simulink model "Expriment_Pose"  (R2014a)
settings: Solver=FixedStepDiscrete  SolverMode=SingleTasking  StartTime=0.0  StopTime=inf  FixedStep=0.01  RelTol=1e-3
PostLoadFcn:
  | h_RPStest = RPStest;
model workspace (MAT data in the model file):
  gtest = 0
undefined symbols (not defined in the file or in its folder): avert, avert_freq_factor, avert_gaze_dirs_chance, avert_gaze_duration_factor, avert_head_frequency_factor, avert_head_speed, BML, BML1, BML2, bmlsL, bmlsM, bodyBusyFlag, clock, emotion_amount_factor, faceBusyFlag, fileID, GAZE_WIN, gazing, mut_freq_factor, mutual_gaze_duration_factor, P, pose_cat_chance, pose_chanc_factor, pose_chance_factor, pose_frequency_factor, pose_lean, pose_lean_flag, pose_speed, pose_twitch, pr, serial, STATE_BEFORE, STATE_GO, STATE_OVER, STATE_READY, Stateflow
libraries: simulink x24, instrumentlib x6, lib_affectiveChar_behavior x2, realtime_pacer_lib x2, lib_affectiveChar_input x1
(part 7 of 7)

== stateflow chart Expriment_Pose/CharacterControl/facialExpression_Controller ==
  state subSmile [parallel]
    settings: executionOrder=1
    state stateInitial
      entry: avert=1; gameState=14;
      n=encStr2Arr(' ');bmlsM=[n n n n n];newBmlsM=[n n n n n];
    state stateCheckSmile
    state gazeCamera
      entry:  [P,BMLM]= smileTable(2) ;avert=0;
      newBmlsM=insertQueue(bmlsM,BMLM);
      bmlsM=newBmlsM;
    state wait
    state checkP
      entry:  [P,BMLM]=  smileTable(1) ;
      newBmlsM=insertQueue(bmlsM,BMLM);
      bmlsM=newBmlsM;
    (default) -> stateInitial
    stateInitial -> stateCheckSmile : [gameState==20]
    stateCheckSmile -> stateCheckSmile [order 2]
    gazeCamera -> stateCheckSmile [order 2] : after(1,secs)[isSmiling~=1]
    wait -> stateCheckSmile : after(10,secs)
    stateCheckSmile -> gazeCamera [order 1] : [[isSmiling==1]&[ gameState~= STATE_GO]&[ gameState~= STATE_READY]]
    checkP -> wait
    gazeCamera -> checkP [order 1] : after(1,secs)[isSmiling==1]
  note: SMILE_DUER=10 seceonds
  note: check if still isSmiling is true works as a buffer to remove the smiles that last ony 1 sec (system errors).
  state subFacial [parallel]
    settings: executionOrder=2
    state stateFacialExpression
      entry:
      emotion_amount_factor =set_AU_Amount(inA,inV,personality);
      BMLl=cmdBML_AU_VA(emotion_amount_factor);
      newBmlsL=insertQueueLow(bmlsL,BMLl); bmlsL=newBmlsL;
    state initial
    state wait3
    (default) -> initial
    initial -> stateFacialExpression : [gameState==20]
    wait3 -> stateFacialExpression : after(7,secs)
    stateFacialExpression -> wait3
  data: bmls function_input double size=[1000,5]; myBML function_input double size=[1000,1]; newBmls function_output double size=[1000,5]; bmls function_input double size=[1000,5]; myBML function_input double size=[1000,1]; newBmls function_output double size=[1000,5]; bmlID function_input double; p function_output double size=1; poseBML function_output double size=[1000,1]; bmlID function_input double; p function_output double size=1; poseBML function_output double size=[1000,1]; eAmountFactor function_output double size=[1,11]; arousal function_input double size=1; valence function_input double size=1; inPersonality function_input double size=1; smileN local double size=1; isSmiling input double size=1 =0; avert data_store_memory =0; gazing data_store_memory size=2; GAZE_WIN data_store_memory size=2; BML data_store_memory size=[256,1]; P data_store_memory; fileID local double size=1; gameState output double; STATE_GO data_store_memory; STATE_READY data_store_memory; STATE_BEFORE data_store_memory; newBmlsM local double size=[1000,5]; bmlsM data_store_memory size=[256,1]; BMLM local double size=[1000,1]; n local; personality input double size=1; internalE input double size=1; au local; emotion_amount_factor data_store_memory; aChange input boolean size=1; au_i local double size=1; au_L local double size=1; emoDisp local; bmlsL data_store_memory size=[256,1]; BMLl local double size=[1000,1]; newBmlsL local double size=[1000,5]; emotion_amount_custom input double size=1; inA input double size=1; inV input double size=1; vChange input boolean size=1
  events: secs input RISING_EDGE_EVENT
  function newBmls =insertQueue(bmls,myBML):
    | function newBmls =insertQueue(bmls,myBML)
    |     full=1;
    |     t=encStr2Arr(' ');
    |     newBmls=[t t t t t];
    |     for i = 1:5
    |         if (isequal(bmls(:,i),t))
    |             %add to end of the queue where its empty
    |             bmls(:,i)=myBML;
    |             full=0;
    |             break
    |         end
    |     end
    |     if(full~=0)
    |             %if queue full, shift all elements to left which removes the first one, then add to end
    |             bmls(:,1)= bmls(:,2);
    |             bmls(:,2)= bmls(:,3);
    |             bmls(:,3)= bmls(:,4);
    |             bmls(:,5)=myBML;
    |     end
    |     newBmls=bmls;
  function newBmls =insertQueueLow(bmls,myBML):
    | function newBmls =insertQueueLow(bmls,myBML)
    |     full=1;
    |     t=encStr2Arr(' ');
    |     newBmls=[t t t t t];
    |     for i = 1:5
    |         if (isequal(bmls(:,i),t))
    |             %add to end of the queue where its empty
    |             bmls(:,i)=myBML;
    |             full=0;
    |             break
    |         end
    |     end
    |     if(full~=0)
    |             %if queue full, shift all elements to left which removes the first one, then add to end
    |             bmls(:,1)= bmls(:,2);
    |             bmls(:,2)= bmls(:,3);
    |             bmls(:,3)= bmls(:,4);
    |             bmls(:,5)=myBML;
    |     end
    |     newBmls=bmls;
  function [p,poseBML] = smileTable(bmlID):
    | function [p,poseBML] = smileTable(bmlID)
    | 
    | aVarTruthTableCondition_1 = false;
    | aVarTruthTableCondition_2 = false;
    | 
    | 
    | % smile
    | 
    | aVarTruthTableCondition_1 = logical(bmlID==1);
    | 
    | % headN
    | 
    | aVarTruthTableCondition_2 = logical(bmlID==2);
    | 
    | if (aVarTruthTableCondition_1)
    |     aFcnTruthTableAction_1();
    | elseif (aVarTruthTableCondition_2)
    |     aFcnTruthTableAction_2();
    | else % Default
    |     aFcnTruthTableAction_1();
    | end
    | 
    | function aFcnTruthTableAction_1()
    | 
    | % smile
    | 
    | poseBML=encStr2Arr('<?xml version="1.0"?><act><bml><face amount="1" au="12" side="BOTH" start="0" stroke="2" relax="3" end="4" type="facs"/><face amount="0.3" au="6" side="BOTH" start="0" stroke="2" relax="3" end="4" type="facs"/></bml></act>');p=3;
    | 
    | function aFcnTruthTableAction_2()
    | 
    | % headNeutralBrow
    | 
    | poseBML=encStr2Arr('<?xml version="1.0" ?><act><bml><gaze target="gazeTarget" start="0" end="5" sbm:time-hint="1.5"/></bml></act>');p=3;
    | 
    | function aFcnTruthTableAction_3()
    | 
    | % smileBrow
    | 
    | poseBML=encStr2Arr('<?xml version="1.0"?><act><bml><face amount="0.1" au="1" side="BOTH" start="0" stroke="2" relax="4" end="6" type="facs"/><face amount="0.1" au="2" side="BOTH" start="0" stroke="2" relax="4" end="6" type="facs"/></bml></act>');p=3;
  function [p,poseBML] = facialExpr(bmlID):
    | function [p,poseBML] = facialExpr(bmlID)
    | 
    | aVarTruthTableCondition_1 = false;
    | aVarTruthTableCondition_2 = false;
    | 
    | 
    | % smile
    | 
    | aVarTruthTableCondition_1 = logical(bmlID==1);
    | 
    | % headN
    | 
    | aVarTruthTableCondition_2 = logical(bmlID==2);
    | 
    | if (aVarTruthTableCondition_1)
    |     aFcnTruthTableAction_1();
    | elseif (aVarTruthTableCondition_2)
    |     aFcnTruthTableAction_2();
    | else % Default
    |     aFcnTruthTableAction_1();
    | end
    | 
    | function aFcnTruthTableAction_1()
    | 
    | % smile
    | 
    | poseBML=encStr2Arr('<?xml version="1.0"?><act><bml><face amount="1" au="12" side="BOTH" start="0" stroke="10" relax="70" end="100" type="facs"/><face amount="0.3" au="6" side="BOTH" start="0" stroke="10" relax="70" end="100" type="facs"/></bml></act>');p=3;
    | 
    | function aFcnTruthTableAction_2()
    | 
    | % headNeutralBrow
    | 
    | poseBML=encStr2Arr('<?xml version="1.0" ?><act><bml><gaze target="gazeTarget" start="0" end="5" sbm:time-hint="1.5"/></bml></act>');p=3;
    | 
    | function aFcnTruthTableAction_3()
    | 
    | % smileBrow
    | 
    | poseBML=encStr2Arr('<?xml version="1.0"?><act><bml><face amount="0.1" au="1" side="BOTH" start="0" stroke="2" relax="4" end="6" type="facs"/><face amount="0.1" au="2" side="BOTH" start="0" stroke="2" relax="4" end="6" type="facs"/></bml></act>');p=3;
  function eAmountFactor  =set_AU_Amount(arousal,valence,inPersonality):
    | function eAmountFactor  =set_AU_Amount(arousal,valence,inPersonality)
    | %     15-12-2015, PAD drivern facial expr simul, Grammer data to map AU and VA
    | %     fprintf('VA: %0.0f,%0.0f\r\n',arousal,valence);
    | %     scale
    | %     p = valence * (20/9)  - 10;
    | %     a = arousal * (20/9)  - 10;
    | 
    |     p=valence;a=arousal;
    |     all_AUs=[1,2,4,5,6, 7,12,26,45,10, 25];eAmountFactor=[0,0,0,0,0, 0,0,0,0,0, 0];
    |     for c=1:11
    |         eAmountFactor(1)=0.003*p-0.002*a;  %1,-0.002*a
    |         eAmountFactor(2)=-0.002*p+0.010*a; %2,+0.010*a
    | %         eAmountFactor(12)=-0.016*p+0.034*a; %27 moth open stretch
    |         eAmountFactor(8)=-0.002*p+0.023*a;  %26,-0.002*p+0.049*a
    |         eAmountFactor(5)=-0.008*p+0.009*a;  %6
    |         
    | %         eAmountFactor(13)=0.002*p+0.004*a; %18 lip Puckerer, W 0.3=101
    | %         eAmountFactor(14)=0.007*p+0.025*a; %22 lip fumeler, ShCh 0.5=102       
    | %         eAmountFactor(15)=0.003*p+0.009*a; %14 dimpler FV+PBM 0.5=103
    | %         eAmountFactor(16)=0.003*p+0.009*a; %14 dimpler FV+PBM 0.5=103
    | %         eAmountFactor=-0.010*p+0.017*a;  %17 chin raiser
    | 
    |         eAmountFactor(10)=-0.020*p+0.020*a;  %10 upper lip raiser,-0.053*p+0.026*a
    |         eAmountFactor(4)=-0.003*p+0.032*a; %5 upper lid raiser
    |         eAmountFactor(9)=-0.011*p-0.011*a; %eye closed, 45 instead of 43,-0.021*p-0.037*a
    |         eAmountFactor(3)=-0.036*p+0.022*a; %4 brow lowerer
    | %       eAmountFactor=-0.008*p+0.006*a;    %9 nose wrikler ,10
    | %       eAmountFactor=-0.004*p+0.004*a;    %39?
    | %       eAmountFactor=-0.010*p+0.008*a;    %38?
    | 
    |         eAmountFactor(11)=-0.011*p+0.023*a;%25 lip open,-0.023*p+0.058*a
    | %       eAmountFactor(17)=-0.004*p-0.003*a;    %24 lip pressor, PBM =104       
    | %       eAmountFactor(18)=-0.011*p+0.009*a;    %23 lip tightner PBM0.2 + W0.6=105
    | %       eAmountFactor(19)=-0.011*p+0.009*a;    %23 lip tightner PBM0.2 + W0.6=105
    | 
    | %       eAmountFactor=-0.004*p+0.003*a;    %19?
    | 
    | %       eAmountFactor(20)=0.039*p+0.015*a;  %13 cheek puffer, W 0.3 =106
    |         
    |         eAmountFactor(6)=-0.005*p-0.001*a; %7  Lid Tightener
    |         eAmountFactor(7)=0.057*p+0.009*a;  %12 Lip Corner Puller
    |     %   eAmountFactor=-0.008*p+0.009*a;    %11 Nasolabial Deepener
    |     %   eAmountFactor=-0.046*p-0.002*a;    %15 Lip Corner Depressor
    |     %   eAmountFactor=-0.014*p+0.016*a;    %16 Lower Lip Depressor
    |     %   eAmountFactor(20)=-0.026*p+0.010*a;%20 lip stretch
    |         
    |         eAmountFactor=eAmountFactor/6; %scale
    |         if(inPersonality==2 || inPersonality==4)%introvert
    |             eAmountFactor=eAmountFactor/1.3; % divide by 4/3
    |         end
    |     end

== stateflow chart Expriment_Pose/GazeFollowSubsystem/reactiveGaze/createGazePawn ==
  state sendBML(In1) [function]
  state sendSBM(In2) [function]
  state stateCreatePawn
    entry:
    sendSBM( encStr2Arr( 'gt = scene.createPawn("gazeTarget")' ) );
    sendBML(encStr2Arr('<?xml version="1.0" ?><act><bml><gaze sbm:joint-range="EYES BACK" target="gazeTarget"/></bml></act>'));
  (default) -> stateCreatePawn
  data: In1 function_input double size=[1000 1]; In2 function_input double size=[1000 1]

== matlab function Expriment_Pose/randomArray/makleArray ==
  data: r1 input; y output double size=[1,25]; r2 input; r3 input; r4 input; r5 input; r6 input; r7 input; r8 input; r9 input; r10 input; r11 input; r12 input; r13 input; r14 input; r15 input; r16 input; r17 input; r18 input; r19 input; r20 input; r21 input; r22 input; r23 input; r24 input; r25 input
function y = fcn(r1,r2,r3,r4,r5,r6,r7,r8,r9,r10,r11,r12,r13,r14,r15,r16, r17, r18, r19,r20,r21,r22,r23,r24,r25)
%#codegen
y=[0,0,0,0,0,0,0,0,0,0,0,0,0,0,0,0,0,0,0,0,0,0,0,0,0];
y(:,1) = floor(r1);
y(:,2) = floor(r2);
y(:,3) = floor(r3);
y(:,4) = floor(r4);
y(:,5) = floor(r5);
y(:,6) = floor(r6);
y(:,7) = floor(r7);
y(:,8) = floor(r8);
y(:,9) = floor(r9);
y(:,10) = floor(r10);
y(:,11) = floor(r11);
y(:,12) = floor(r12);
y(:,13) = floor(r13);
y(:,14) = floor(r14);
y(:,15) = floor(r15);
y(:,16) = floor(r16);
y(:,17) = floor(r17);
y(:,18) = floor(r18);
y(:,19) = floor(r19);
y(:,20) = floor(r20);
y(:,21) = floor(r21);
y(:,22) = floor(r22);
y(:,23) = floor(r23);
y(:,24) = floor(r24);
y(:,25) = floor(r25);

== matlab function Expriment_Pose/facialExpr/checkNeutral ==
  data: notNeutral output double size=1; e input
function notNeutral = fcn(e)
%#codegen

if(e~=6)
    notNeutral=1;
else
    notNeutral=0;
end

== stateflow chart Expriment_Pose/CharacterControl/wave_Controller ==
  state init
    entry: STATE_OVER=3;
    STATE_BEFORE=4;
    gameState=14;
    rFlag=0;lFlag=0;bFlag=0;
    n=encStr2Arr(' ');bmlsM=[n n n n n];
    newBmlsM=[n n n n n];
  state waveRightHand
    entry: [P,BMLM]= wavePoseBradTable(1+animNum);
    rFlag=1;
    newBmlsM=insertQueue(bmlsM,BMLM);
    bmlsM=newBmlsM;
  state gazeCamera
    entry: [P,BMLM]= wavePoseBradTable(8);
    avert=0;
    newBmlsM=insertQueue(bmlsM,BMLM);
    bmlsM=newBmlsM;
  state wave
    entry: animNum =setPersonalityParams(personality);
  state waveLeftHand
    entry:
    [P,BMLM]= wavePoseBradTable(animNum);
    lFlag=1;
    newBmlsM=insertQueue(bmlsM,BMLM);
    bmlsM=newBmlsM;
  state gazeCamera1
    entry: [P,BMLM]= wavePoseBradTable(8);
    avert=0;
    newBmlsM=insertQueue(bmlsM,BMLM);
    bmlsM=newBmlsM;
  note: if introvert 50% chance of introvertWave(poseN=7)
  note: else(extrovert)
  state gazeCamera2
    entry: [P,BMLM]= wavePoseBradTable(8);
    avert=0;
    newBmlsM=insertQueue(bmlsM,BMLM);
    bmlsM=newBmlsM;
  state waveBothHands
    entry: [P,BMLM]= wavePoseBradTable(3+animNum);
    bFlag=1;
    newBmlsM=insertQueue(bmlsM,BMLM);
    bmlsM=newBmlsM;
  note: Problem with procedural behaviors (you can not give duration and they stay in that pose untill new bml comes so they dont return to idle)
      | we want the agent to gaze at user for the period of waving.If new idle gaze BML comes, agent averts gaze or head before wave finished. Gaze is procedural (gazes at the point till new gaze bml is recieved so it does not automatically return to idle pose) so we can not give duration of gaze in the BML. The only way to avoid avert during wave is to make sure thre is no idle gaze bmls during the wave; which makes sense considering the gaze does not avert(idle) when you are attending something.
      | prioritizing does not solve this because avertGaze comes right after gazeCamera and wave. We also can not delay after high priorities because sometime several high priorities should happen right after eachother.
  waveBothHands -> wave : after(5,secs)
  waveRightHand -> wave : after(5,secs)
  waveLeftHand -> wave : after(5,secs)
  (default) -> init
  init -> wave
  (junction 55) -> waveRightHand [order 2]
  gazeCamera -> waveRightHand : after(2,secs)
  wave -> (junction 55) [order 4] : [[handUp==1]&[rFlag==0]]{ lFlag=0;bFlag=0;}
  (junction 55) -> gazeCamera [order 1] : [avert==1]
  wave -> wave [order 1] : after(10,secs){ rFlag=0;lFlag=0;bFlag=0;}
  wave -> (junction 59) [order 3] : [[handUp==3]&[bFlag==0]]{ rFlag=0;lFlag=0;}
  wave -> (junction 58) [order 2] : [[handUp==2]&[lFlag==0]]{ rFlag=0;bFlag=0;}
  (junction 82) -> waveLeftHand [order 1] : [randP==1]{animNum=7;}
  (junction 58) -> (junction 79) [order 2]
  (junction 79) -> (junction 82) [order 1] : [[personality==2]|[personality==4]]{randP=randArray(:,12)}
  (junction 58) -> gazeCamera1 [order 1] : [avert==1]
  gazeCamera1 -> (junction 79) : after(2,secs)
  (junction 79) -> waveLeftHand [order 2] : {animNum=2+animNum;}
  (junction 82) -> waveLeftHand [order 2] : [randP==2]{animNum=2+animNum;}
  (junction 59) -> waveBothHands [order 2]
  (junction 59) -> gazeCamera2 [order 1] : [avert==1]
  gazeCamera2 -> waveBothHands : after(2,secs)
  data: pr function_output double size=1; bmlID function_input double; poseBML function_output double size=[1000,1]; num function_output double size=1; p function_input double size=1; bmls function_input double size=[1000,5]; mBML function_input double size=[1000,1]; newBmls function_output double size=[1000,5]; fileID data_store_memory; handUp input; gameState output double size=1; BML data_store_memory; P data_store_memory; STATE_OVER data_store_memory; STATE_BEFORE data_store_memory; rFlag local; lFlag local; bFlag local; BML2 data_store_memory; avert data_store_memory; BMLM local double size=[1000,1]; newBmlsM local double size=[1000,5]; bmlsM data_store_memory; n local; personality input double size=1; randP local; animNum local; randArray input double size=[1,25]; personalityChange input boolean size=1
  events: secs input RISING_EDGE_EVENT
  function [pr,poseBML]=wavePoseBradTable(bmlID):
    | function [pr,poseBML]=wavePoseBradTable(bmlID)
    | 
    | aVarTruthTableCondition_1 = false;
    | aVarTruthTableCondition_2 = false;
    | aVarTruthTableCondition_3 = false;
    | aVarTruthTableCondition_4 = false;
    | aVarTruthTableCondition_5 = false;
    | aVarTruthTableCondition_6 = false;
    | aVarTruthTableCondition_7 = false;
    | aVarTruthTableCondition_8 = false;
    | aVarTruthTableCondition_9 = false;
    | aVarTruthTableCondition_10 = false;
    | 
    | 
    | 
    | aVarTruthTableCondition_1 = logical(bmlID==1);
    | 
    | 
    | aVarTruthTableCondition_2 = logical(bmlID==2);
    | 
    | 
    | aVarTruthTableCondition_3 = logical(bmlID==3);
    | 
    | 
    | aVarTruthTableCondition_4 = logical(bmlID==4);
    | 
    | 
    | aVarTruthTableCondition_5 = logical(bmlID==5);
    | 
    | 
    | aVarTruthTableCondition_6 = logical(bmlID==6);
    | 
    | 
    | aVarTruthTableCondition_7 = logical(bmlID==7);
    | 
    | 
    | aVarTruthTableCondition_8 = logical(bmlID==8);
    | 
    | 
    | aVarTruthTableCondition_9 = logical(bmlID==9);
    | 
    | 
    | aVarTruthTableCondition_10 = logical(bmlID==10);
    | 
    | if (aVarTruthTableCondition_1)
    |     aFcnTruthTableAction_1();
    | elseif (aVarTruthTableCondition_2)
    |     aFcnTruthTableAction_2();
    | elseif (aVarTruthTableCondition_3)
    |     aFcnTruthTableAction_3();
    | elseif (aVarTruthTableCondition_4)
    |     aFcnTruthTableAction_4();
    | elseif (aVarTruthTableCondition_5)
    |     aFcnTruthTableAction_5();
    | elseif (aVarTruthTableCondition_6)
    |     aFcnTruthTableAction_6();
    | elseif (aVarTruthTableCondition_7)
    |     aFcnTruthTableAction_7();
    | elseif (aVarTruthTableCondition_8)
    |     aFcnTruthTableAction_8();
    | elseif (aVarTruthTableCondition_9)
    |     aFcnTruthTableAction_9();
    | elseif (aVarTruthTableCondition_10)
    |     aFcnTruthTableAction_10();
    | else % Default
    |     aFcnTruthTableAction_1();
    | end
    | 
    | function aFcnTruthTableAction_1()
    | 
    | % waveLeftF
    | 
    | poseBML=encStr2Arr('<?xml version="1.0" ?><act><bml><animation name="../data/ChrBrad/test_wave_left.skm" speed="2"/></bml></act>'); pr=2;
    | 
    | function aFcnTruthTableAction_2()
    | 
    | % waveRightF
    | 
    | poseBML=encStr2Arr('<?xml version="1.0" ?><act><bml><animation name="../data/ChrBrad/test_wave_right.skm" speed="2"/></bml></act>'); pr=2;
    | 
    | function aFcnTruthTableAction_3()
    | 
    | % waveBothF
    | 
    | poseBML=encStr2Arr('<?xml version="1.0" ?><act><bml><animation name="ChrBrad@Idle01_BeatHighBt01" speed="2"/></bml></act>'); pr=2;
    | 
    | function aFcnTruthTableAction_4()
    | 
    | % waveLeftSlow
    | 
    | poseBML=encStr2Arr('<?xml version="1.0" ?><act><bml><animation name="../data/ChrBrad/test_wave_left.skm" speed="0.5"/></bml></act>'); pr=2;
    | 
    | function aFcnTruthTableAction_5()
    | 
    | % WaveRightSlow
    | 
    | poseBML=encStr2Arr('<?xml version="1.0" ?><act><bml><animation name="../data/ChrBrad/test_wave_right.skm" speed="0.5"/></bml></act>'); pr=2;
    | 
    | function aFcnTruthTableAction_6()
    | 
    | % WaveBothSlow
    | 
    | poseBML=encStr2Arr('<?xml version="1.0" ?><act><bml><animation name="ChrBrad@Idle01_BeatHighBt01" speed="0.5"/></bml></act>'); pr=2;
    | 
    | function aFcnTruthTableAction_7()
    | 
    | % WaveLIntrovert
    | 
    | poseBML=encStr2Arr('<?xml version="1.0" ?><act><bml><animation name="../data/ChrBrad/test_introvert_wave.skm" speed="1"/></bml></act>'); pr=2;
    | 
    | function aFcnTruthTableAction_8()
    | 
    | % gazeCamera
    | 
    | poseBML=encStr2Arr('<?xml version="1.0" ?><act><bml><gaze target="gazeTarget" sbm:joint-range="EYES NECK" sbm:time-hint="1.5"/></bml></act>');pr=2;
    | 
    | function aFcnTruthTableAction_9()
    | 
    | % waveLeft
    | 
    | poseBML=encStr2Arr('<?xml version="1.0" ?><act><bml><animation name="ChrBrad@Idle01_BeatHighRt01"/></bml></act>');pr=2;
    | 
    | function aFcnTruthTableAction_10()
    | 
    | % waveRight
    | 
    | poseBML=encStr2Arr('<?xml version="1.0" ?><act><bml><animation name="ChrBrad@Idle01_BeatHighRt01"/></bml></act>');pr=2;
  function num =setPersonalityParams(p):
    | function num =setPersonalityParams(p)
    |  num=0;
    |  if(p==1) %HE
    |     num=0;
    |  elseif(p==2)%LE
    |     num=3;
    |  elseif(p==3)%HE
    |     num=0;
    |  else%LE
    |     num=3;
    |  end
  function newBmls =insertQueue(bmls,mBML):
    | function newBmls =insertQueue(bmls,mBML)
    |     full=1;
    |     t=encStr2Arr(' ');
    |     newBmls=[t t t t t];
    |     for i = 1:5
    |         if (isequal(bmls(:,i),t))
    |             %add to end of the queue where its empty
    |             bmls(:,i)=mBML;
    |             full=0;
    |             break
    |         end
    |     end
    |     if(full~=0)
    |             %if queue full, shift all elements to left which removes the first one, then add to end
    |                         disp('before add when full');disp(bmls);
    |             bmls(:,1)= bmls(:,2);
    |             bmls(:,2)= bmls(:,3);
    |             bmls(:,3)= bmls(:,4);
    |             bmls(:,5)=mBML;
    |             
    |     end
    |     newBmls=bmls;

== matlab function Expriment_Pose/facialExpr/facialExprGen/matlabFuncIf/reset ==
  data: L input; u1 input; y output
function y = fcn(L,u1)
if(u1<=L)
    y= u1;
else
    y =1;
end

== matlab function Expriment_Pose/facialExpr/facialExprGen/matlabFuncIf/displayBMLs ==
  data: e input; l input; i input double size=1 [1..]; bml input
function fcn(e,l,i,bml)
%#codegen
fprintf('%s','e:');fprintf('%f',e);
fprintf('%s','  ,L:');fprintf('%f',l);
fprintf('%s','  ,i:');fprintf('%f',i);
disp(decArr2Str(bml));

== matlab function Expriment_Pose/facialExpr/facialExprGen/matlabFuncIf/plusOne ==
  data: y output; i input double size=1
function y  = iCheck(i)
%#codegen
    y=i+1;

== matlab function Expriment_Pose/facialExpr/facialExprGen/matlabFuncIf/makeBmls ==
  data: i input double size=1 [1..]; arrAU input; eAmount input; arrBML output
function arrBML = fcn(i,arrAU,eAmount)
    %#codegen
    coder.extrinsic('sprintf');
    coder.extrinsic('strcat');
    
    %Maryam, 14-10-2015
    %'strcat' dimension 2  maximum size is 453,it was not possible to concat and send all bmls 
    %for one emotion together(used simulink for loop )    
    
    AU=arrAU(i);eA=eAmount(i);   
    c1 = countDigits(AU);c2 = countDigits(eA);

    str1 = sprintf('<?xml version=\"1.0\" ?><act><bml>');
    
    if(max(ceil(log10(abs(AU))),1)==1) %if AU is one-digit
        temp = sprintf('<face type=\"FACS\" side=\"BOTH\" au=\"%1d\"  start=\"0\" ready=\"1\" stroke=\"2\"  relax=\"300\" end=\"400\" amount=\"%0.1f\"/>',AU,eA); 
        temp2=strcat(str1,temp);
        str1=temp2;
    else      
        temp = sprintf('<face type=\"FACS\" side=\"BOTH\" au=\"%2d\" start=\"0\" ready=\"1\" stroke=\"2\"  relax=\"300\" end=\"400\" amount=\"%0.1f\"/>',AU,eA);
        temp2=strcat(str1,temp);
        str1=temp2;
    end

    str2 = sprintf('</bml></act>');
    %n=length(arrAU);
    %mystr=blanks(arrAU(n));
    mystr=blanks(142+c1+c2);
    mystr = strcat (str1,str2);    
    arrBML = encStr2Arr(mystr);

== matlab function Expriment_Pose/facialExpr/facialExprGen/forloop1/makeBmls ==
  data: i input double size=1 [1..]; arrAU input; eAmount input; arrBML output
function arrBML = fcn(i,arrAU,eAmount)
    %#codegen
    coder.extrinsic('sprintf');
    coder.extrinsic('strcat');
    
    %Maryam, 14-10-2015
    %'strcat' dimension 2  maximum size is 453,it was not possible to concat and send all bmls 
    %for one emotion together(used simulink for loop )    
    
    AU=arrAU(i);eA=eAmount(i);   
    c1 = countDigits(AU);c2 = countDigits(eA);

    str1 = sprintf('<?xml version=\"1.0\" ?><act><bml>');
    
    if(max(ceil(log10(abs(AU))),1)==1) %if AU is one-digit
        temp = sprintf('<face type=\"FACS\" side=\"BOTH\" au=\"%1d\"  start=\"0\" ready=\"1\" stroke=\"2\"  relax=\"3\" end=\"4\" amount=\"%0.1f\"/>',AU,eA); 
        temp2=strcat(str1,temp);
        str1=temp2;
    else      
        temp = sprintf('<face type=\"FACS\" side=\"BOTH\" au=\"%2d\" start=\"0\" ready=\"1\" stroke=\"2\"  relax=\"3\" end=\"4\" amount=\"%0.1f\"/>',AU,eA);
        temp2=strcat(str1,temp);
        str1=temp2;
    end

    str2 = sprintf('</bml></act>');
    %n=length(arrAU);
    %mystr=blanks(arrAU(n));
    mystr=blanks(140+c1+c2);
    mystr = strcat (str1,str2);    
    arrBML = encStr2Arr(mystr);

== matlab function Expriment_Pose/EmotionSubsystem/calculateValenceArousal/HELN_VA_Emo ==
  data: V input; e output double size=1; A input double
function e = fcn(V, A)

aVarTruthTableCondition_1 = false;
aVarTruthTableCondition_2 = false;
aVarTruthTableCondition_3 = false;
aVarTruthTableCondition_4 = false;
aVarTruthTableCondition_5 = false;
aVarTruthTableCondition_6 = false;
aVarTruthTableCondition_7 = false;
aVarTruthTableCondition_8 = false;


% 7-happy  2,1

aVarTruthTableCondition_1 = logical(V>10 && A<40 && A>10);

% 8-ex  1,2 AND 2,2

aVarTruthTableCondition_2 = logical(V>0 && A>40);

% 4-fear  -1,2 AND -2,2

aVarTruthTableCondition_3 = logical(V<0 && A>40);

% 3-frust  -2,1

aVarTruthTableCondition_4 = logical(V<-10 && A<40 && A>10);

% 6-idle  2,-1

aVarTruthTableCondition_5 = logical(V>10 && A<-10 && A>-40);

% 5-calm  1,-2 AND 2,-2

aVarTruthTableCondition_6 = logical(V>0 && A<-40);

% 1-bored  -1,-2 AND -2,-2

aVarTruthTableCondition_7 = logical(V<0 && A<-40);

% 2-sad  -2,-1

aVarTruthTableCondition_8 = logical(V<-10 && A<-10 && A>-40);

if (aVarTruthTableCondition_1)
    aFcnTruthTableAction_1();
elseif (aVarTruthTableCondition_2)
    aFcnTruthTableAction_2();
elseif (aVarTruthTableCondition_3)
    aFcnTruthTableAction_3();
elseif (aVarTruthTableCondition_4)
    aFcnTruthTableAction_4();
elseif (aVarTruthTableCondition_5)
    aFcnTruthTableAction_5();
elseif (aVarTruthTableCondition_6)
    aFcnTruthTableAction_6();
elseif (aVarTruthTableCondition_7)
    aFcnTruthTableAction_7();
elseif (aVarTruthTableCondition_8)
    aFcnTruthTableAction_8();
else % Default
    aFcnTruthTableAction_5();
end

function aFcnTruthTableAction_1()

% happy

e=7;

function aFcnTruthTableAction_2()

% excited

e=8;

function aFcnTruthTableAction_3()

% fear

e=4;

function aFcnTruthTableAction_4()

% frustration

e=3;

function aFcnTruthTableAction_5()

% idle

e=6;

function aFcnTruthTableAction_6()

% contempt

e=5;

function aFcnTruthTableAction_7()

% bored

e=1;

function aFcnTruthTableAction_8()

% sad

e=2;

== stateflow chart Expriment_Pose/CharacterControl/personality_Behavior_Factors ==
  state setP
    entry:
    %[mutual_gaze_duration_factor, avert_gaze_duration_factor,avert_head_frequency_factor,avert_head_speed,avert_gaze_dirs_chance,avert_freq_factor,mut_freq_factor,blink_flag, blinkperiod_min,blinkperiod_max]=sharedFunc.setGazeFactors(inV,inA,personality,personalityFlag,vaFlag,gazeArray);
    [pose_twitch,pose_frequency_factor,pose_chanc_factor,pose_cat_chance,pose_lean,pose_speed,pose_lean_flag]=sharedFunc.setPoseFactors(inV,inA,personality,personalityFlag,vaFlag,poseArray,personalityChange);
  state init
    entry: mutual_gaze_duration_factor=1;avert_gaze_duration_factor=1;,avert_freq_factor=1;mut_freq_factor=1;
    avert_head_frequency_factor=20;avert_head_speed=1;avert_gaze_dirs_chance=1;blink_flag=0; blinkperiod_min=5;blinkperiod_max=9;
    pose_lean_flag=0; pose_frequency_factor=20;pose_chanc_factor=1;pose_cat_chance=70;pose_lean=10;pose_speed=1;
  state wait
  state sharedFunc [group]
  (default) -> init
  setP -> wait
  wait -> setP : [personalityChange==1]
  init -> wait
  data: inA input double size=1; inV input double size=1; vaFlag input boolean size=1; personalityFlag input boolean size=1; gazeArray input double size=[1, 6]; personality input double size=1; personalityChange input boolean size=1; mutual_gaze_duration_factor data_store_memory; avert_head_frequency_factor data_store_memory; avert_gaze_duration_factor data_store_memory; avert_head_speed data_store_memory; avert_gaze_dirs_chance data_store_memory; poseArray input double size=[1, 6]; pose_chanc_factor data_store_memory; pose_frequency_factor data_store_memory; pose_lean data_store_memory; pose_change_flag data_store_memory; pose_lean_flag data_store_memory; pose_speed data_store_memory; pose_cat_chance data_store_memory; internalE input double size=1; emotion_amount_custom input double size=1; emotion_amount_factor data_store_memory size=1; mut_freq_factor data_store_memory; avert_freq_factor data_store_memory; pose_twitch data_store_memory; blinkperiod_min data_store_memory; blink_flag data_store_memory; blinkperiod_max data_store_memory

== stateflow chart Expriment_Pose/CharacterControl/custom_Behavior_Factors ==
  state setP
    entry:
    [mutual_gaze_duration_factor, avert_gaze_duration_factor,avert_head_frequency_factor,avert_head_speed,avert_gaze_dirs_chance,avert_freq_factor,mut_freq_factor]=sharedFunc.setGazeFactors(inV,inA,personality,personalityFlag,vaFlag,gazeArray);
  state init
    entry: mutual_gaze_duration_factor=1;avert_gaze_duration_factor=1;
    avert_head_frequency_factor=1;avert_head_speed=1;avert_gaze_dirs_chance=1;,avert_freq_factor=1;mut_freq_factor=1;
    pose_frequency_factor=5;pose_chanc_factor=1;pose_cat_chance=10;pose_lean=10;pose_speed=1;pose_lean_flag=0;
  state wait
  state sharedFunc [group]
  state setP1
    entry:
    [pose_twitch,pose_frequency_factor,pose_chanc_factor,pose_cat_chance,pose_lean,pose_speed,pose_lean_flag]=sharedFunc.setPoseFactors(inV,inA,personality,personalityFlag,vaFlag,poseArray,personalityChange);
  (default) -> init
  init -> wait
  setP -> wait
  wait -> setP [order 1] : [gazeArray(:,1)==1]
  setP1 -> wait
  wait -> setP1 [order 2] : [poseArray(:,1)==1]
  data: inA input double size=1; inV input double size=1; vaFlag input boolean size=1; personalityFlag input boolean size=1; gazeArray input double size=[1, 6]; personality input double size=1; personalityChange input boolean size=1; mutual_gaze_duration_factor data_store_memory; avert_head_frequency_factor data_store_memory; avert_gaze_duration_factor data_store_memory; avert_head_speed data_store_memory; avert_gaze_dirs_chance data_store_memory; poseArray input double size=[1, 6]; pose_lean data_store_memory; pose_speed data_store_memory; pose_chanc_factor data_store_memory; pose_frequency_factor data_store_memory; pose_cat_chance data_store_memory; pose_lean_flag data_store_memory; emotion_amount_custom input double size=1; emotion_amount_factor data_store_memory size=1; mut_freq_factor data_store_memory; avert_freq_factor data_store_memory; pose_twitch data_store_memory

== matlab function Expriment_Pose/EmotionSubsystem/calculateValenceArousal/HELN plot ==
  data: v input; a input
function fcn(v,a)
%coder.extrinsic to bypass code generation
coder.extrinsic('fscanf')
coder.extrinsic('get_param');
% coder.extrinsic('importdata');

currentTime=get_param('Expriment_FacialExpr','SimulationTime');%use name of simulink proj

A = [v;a;currentTime];

fileID = fopen('HELN_VA_table.txt','a');
fprintf(fileID,'%0.1f,%0.1f,%0.1f\r\n',A);
fclose(fileID);

%use the following to draw the plot
%tmp_data = importdata('HEHN_VA_table.txt',','); 
%no need: x=tmp_data(:,1);y=tmp_data(:,2);z=tmp_data(:,3)
%matrix=tmp_data
%tri = delaunay(matrix(:,1),matrix(:,2));
%trisurf(tri,matrix(:,1),matrix(:,2),matrix(:,3))
%shading interp

%-----------------------------------------
% fileID = fopen('HEHN_VA_table.txt','r');
% formatSpec = '%1f\r %1f\r %1f\r\n';
% sizeA = [3 Inf];
% A = fscanf(fileID,formatSpec,sizeA)
% % A = A'
% fclose(fileID);

% x = zeros(100,2);y = zeros(100,2);
% filename = 'HEHN_VA_table.txt';
% delimiterIn = ' ';
% headerlinesIn = 1;
% A = importdata(filename,delimiterIn,headerlinesIn);

% fileID=fopen('HEHN_VA_table4.txt');
% s=textscan(fileID,'%d %d %d','headerlines',23);
% fclose(fileID);
% x=s{1}

== matlab function Expriment_Pose/CharacterControl/personality_Behavior_Factors/sharedFunc ==
  data: v function_input double size=1; a function_input double size=1; mutDurFactor function_output double size=1; avertDurFactor function_output double size=1; avertHeadFreqFactor function_output double size=1; p function_input double size=1; pFlag function_input boolean size=1; vaFlag function_input boolean size=1; avertHeadSpeed function_output double size=1; gazeArr function_input double size=[1,6]; avertDirsChance function_output double size=1; avertFreqFactor function_output double size=1; mutFreqFactor function_output double size=1; blinkFlag function_output double size=1; blinkPeriodMin function_output double size=1; blinkPeriodMax function_output double size=1; poseTwitch function_output double size=1; poseFreqFactor function_output double size=1; poseChanceFactor function_output double size=1; poseCatChance function_output double size=1; poseLean function_output double size=1; v function_input double size=1; ar function_input double size=1; p function_input double size=1; pFlag function_input boolean size=1; vaFlag function_input boolean size=1; poseSpeed function_output double size=1; poseArr function_input double size=[1,6]; poseLeanFlag function_output double size=1; personalityChange function_input double size=1
function [mutDurFactor,avertDurFactor,avertHeadFreqFactor,avertHeadSpeed,avertDirsChance,avertFreqFactor,mutFreqFactor,blinkFlag,blinkPeriodMin,blinkPeriodMax]=setGazeFactors(v,a,p,pFlag,vaFlag,gazeArr)
    % Valence/Arousal: ref?
    %V+A+ (excite,happy):high mutual dur,head avert freq less,high freq of change btw mut/avert(MMMMMMMAAMMMMMAMMMA)
    %V-A+ (fear,frust): mid mut/avert,,head avert freq mid,high freq of change btw mut/avert(MMAAMMMAAMMAAAMMMAAAMA)
    %V+A- (idle, calm): mid mut/avert,head avert freq mid,low freq of change btw mut/avert(MMMMMMMAAAAAAMMMMMAAAAA)
    %V-A- (bored,sad):  avert dur more,,head avert freq more,,high freq of change btw mut/avert(AAAAAAMAAAAAAAAMAAAAA)
    %V+A+: v>0 & a>0,V-A+: v<0 & a>0,V+A-:v>0 & a<0,V-A-:v<0 & a<0

    %paper: Effects of Direct and Averted Gaze on the Perception of Facially Communicated Emotion
    % rate of approach-oriented dispositions (i.e., anger and joy) higher for direct relative gaze stimuli
    %avoidance-oriented dispositions (i.e., fear and sadness) would be higher for averted gaze faces.

    %russel, mehrabian circumplex:
    % v-mid,a-mid:approach;     v-mid,a+:avoid;       v-mid,a-:avoid
    % v+,a-mid:mid-approach;    v+,a+:high-approach;  v+,a-:low-approach
    % v-,a-mid:mid-avoid;        v-,a+:high-avoid;    v-,a-:low-avoid

    % marsella, emotional gaze:
    % a+:high blink, faster move
    
    %PERSONALITY:
    % HEHN:mutual dur more,head avert freq more,high freq of change btw mut/avert(MAMAMMAMMMAMAMMAMMAMA)
    % LEHN:avert dur  more,head avert freq more, high freq of change btw mut/avert(AMAAMAAAMAMAAAMAAMAAM)
    % HELN:mutual dur  more,head avert freq less,low freq of change btw mut/avert(MMMMMMMAMMMMMMMMAMMM)
    % LELN:avert  dur more,head avert freq more,low freq of change btw mut/avert(AAAAAAMAAAAAAAAMAAAAA)
    
    %Perception of personality through eye gaze, Ruhland et al
    %Extravert: gaze tward,long,often,up-center-left-right; few blinks ; wide fast node
    %Introvert: gaze Avoidance,short,seldom,down-center; normal blinks; small slow node
    %Neurotic: gaze Avoidance,short,seldom,down-left-right; often blinks; None
    %Stable: gaze tward,medium,medium,center-left-right; normal blinks ; None
    
    %Saccadic reaction time is between 0.18sec and 0.22sec on average.Minimum intersaccadic interval ranges from 0.05sec to 0.1sec
    %smartbody DOF:magnitude:~btw 5'&12'->chanceO:btw 3&8->aveDur:btw 0.26sec&0.18sec --> 
    %simulation sample time is 0.001 so btw 26 and 18
    %magnitude=-6.9*log(chanceO/15.7) -->  -6.9*log(3/15.7)=11.4,-6.9*log(8/15.7)=4.6
    %chanceO=randArray(:,7)-->(3,8); 
    %avertDur=(25+2.5*magnitude)/2*factor;(same for mutual):btw(25+2.5*11.4)/2=26,(25+2.5*4.6)/2=18
    %randHeadChance=randi([1,1+round(randArray(3,5)/avert_head_frequency_factor)]);

    mutDurFactor=1; 
    avertDurFactor=1;  
    avertHeadFreqFactor=20;
    avertHeadSpeed=1;%1=normal, 2=fast&up,3=slow&down
    avertDirsChance=0;%not 1 & 2 is normal
    avertFreqFactor=1;
    mutFreqFactor=1;
    blinkFlag=0;
    blinkPeriodMin=5.0; %normal
    blinkPeriodMax=9.0;%normal

    if(pFlag==1)
        if(p==1)%HEHN  %HE few blinks,HN often blinks
            mutDurFactor=2; % HEHN mut longer ,HN freq more, mutDur=((25+2.5*magnitude)*mutual_gaze_duration_factor)/7;
            avertDurFactor=0.5;  %HE avert less, avertDur=((25+2.5*magnitude)*avert_gaze_duration_factor)/7;
            avertHeadFreqFactor=30;%HE avert head more, randHeadChance=randi([1,1+round(randArray(:,3)/avert_head_frequency_factor)]);
            avertHeadSpeed=2;%HE fast&up, headSpeed={1,2,3}
            avertDirsChance=1;%HE up
            
            mutFreqFactor=3;
            avertFreqFactor=0.5;
            
            blinkFlag=1;
            blinkPeriodMin=0.2; %often
            blinkPeriodMax=7.0;%few
        elseif(p==2) %LEHN %LE normal blinks, HN often blinks
            mutDurFactor=0.5; % LE mut less(mutDur/10) ,HN freq more
            avertDurFactor=2; % (avertDur/4)
            avertHeadFreqFactor=15;%LE avert head less
            avertHeadSpeed=3;%LE slow&down
            avertDirsChance=2;%LE down
            
            mutFreqFactor=0.5;
            avertFreqFactor=3;
            
            blinkFlag=1;
            blinkPeriodMin=0.2; %often
            blinkPeriodMax=5.0;%norm
        elseif(p==3) %HELN %HE few blinks, LN normal blinks 
            mutDurFactor=4; % HE dur more, LN freq less
            avertDurFactor=0.1; % /4 
            avertHeadFreqFactor=25;%HE avert head more
            avertHeadSpeed=2;%fast
            avertDirsChance=1;%HE up
            
            mutFreqFactor=3;
            avertFreqFactor=0.5;
            
            blinkFlag=1;
            blinkPeriodMin=5.0; %normal
            blinkPeriodMax=15.0;%few
        else %LELN %LE normal blinks, LN normal blinks 
            mutDurFactor=0.25; % /4 
            avertDurFactor=0.5;% /2 
            avertHeadFreqFactor=10;%LE avert head less
            avertHeadSpeed=3;%slow
            avertDirsChance=2;%LE down
            
            mutFreqFactor=0.5;
            avertFreqFactor=3;
            
            blinkFlag=1;
            blinkPeriodMin=5.0; %normal
            blinkPeriodMax=9.0;%normal
        end  
    end
    
    if(vaFlag==1)
        if(v>40 && a>40)%V+A+,high-approach,mutual alot
            mutDurFactor=mutDurFactor*2; % /2
            avertDurFactor=round(avertDurFactor*0.5);  % /2
            avertHeadFreqFactor=round(avertHeadFreqFactor/3);%high-approach:head not avert
            avertHeadSpeed=2;%aroused fast
            blinkFlag=1;
            %27-12-2015- Best way to set the blink period is as a linear function of arousal amount
            %      val/(1+((2-1)*(A/100))) 
            %in which val is BlinkMin or BlinkMax and A is arousal amount; this function sets the
            %blinkPriodMin and max to half for twice blink in arousal=100 and to their default at 
            %arousal=1 sicne we need to re-calculate and send sbms continiously I avoided that for 
            % now, instead I only increase min and max when Arousal passes 50 threshold
            blinkPeriodMin=blinkPeriodMin/2; %often
            blinkPeriodMax=blinkPeriodMax/2;

        elseif(v<-40 && a>40) %V-A+,high-avoid, avert alot
            mutDurFactor=round(mutDurFactor*0.5); % /2
            avertDurFactor=avertDurFactor*2; % /2
            avertHeadFreqFactor=avertHeadFreqFactor+30;%high-avoid:head avert alot
            avertHeadSpeed=2;%fast
            blinkFlag=1;
            blinkPeriodMin=blinkPeriodMin/2; %often
            blinkPeriodMax=blinkPeriodMax/2;

        elseif(v>40 && a<-40) %V+A- ,low-approach, mutual most
            mutDurFactor=round(mutDurFactor*1.5); %  /2
            avertDurFactor=round(avertDurFactor*0.75); %/2
            avertHeadFreqFactor=round(avertHeadFreqFactor/2);%approach:head not avert
            avertHeadSpeed=1;%slow&down

        elseif(v<-40 && a<-40) %V-A-,  low-avoid, avert most
            mutDurFactor=round(mutDurFactor*0.75); %/2
            avertDurFactor=round(avertDurFactor*1.5);% /2
            avertHeadFreqFactor=avertHeadFreqFactor+20;%avoid:head avert alot
            avertHeadSpeed=1;%slow&down
        end
    
        
    end

== matlab function Expriment_Pose/CharacterControl/personality_Behavior_Factors/sharedFunc ==
function [poseTwitch,poseFreqFactor,poseChanceFactor,poseCatChance,poseLean,poseSpeed,poseLeanFlag]=setPoseFactors(v,ar,p,pFlag,vaFlag,poseArr,personalityChange)   
    
    pose_custom_flag=poseArr(:,1);
    pose_chance_custom=poseArr(:,3);
    pose_selfAdaptor_chance_custom=poseArr(:,2);
    pose_frequency_custom=poseArr(:,4);
    pose_speed_custom=poseArr(:,5);
    pose_lean_custom=poseArr(:,6);

    poseCatChance=70;
    poseChanceFactor=1;
    poseFreqFactor=20;
    poseSpeed=0;%1=normal;2=fast; 3=slow;
    poseLean=10;
    poseTwitch=0;
    poseLeanFlag=0;

    if(pose_custom_flag==0)    
        if(pFlag==1)
            if(personalityChange==1)
                poseLeanFlag=1;
            end
            if(p==1) %HEHN
                 poseTwitch=1;%HN
                 poseFreqFactor=10;%HN more freq,after(pose_frequency_factor,secs)
                 poseLean=11;
                 poseChanceFactor=2;% HE high chance,randPoseChance=randi([0,round(interest*randSlowPose/pose_chance_factor)]);
                 poseCatChance=90;%HN high selfA,[randPR<=pose_selfAdaptor_chance_factor ]
                 poseSpeed=2;%fast
             elseif(p==2)%LEHN
                 poseTwitch=1;%HN
                 poseFreqFactor=17;%LEHN more freq but low speed
                 poseLean=12;
                 poseChanceFactor=1;%LE less chance
                 poseCatChance=10;%HN high:90% adaptor
                 poseSpeed=3;%slow
             elseif(p==3)%HELN
                 poseTwitch=0;%LN
                 poseFreqFactor=12;%HELN low chance
                 poseLean=11;
                 poseChanceFactor=2;%HE high chance
                 poseCatChance=10;%  10% adapter
                 poseSpeed=2;
             else%LELN
                 poseTwitch=0;%LN
                 poseFreqFactor=20;
                 poseLean=12;
                 poseChanceFactor=1;%LE low chance
                 poseCatChance=90;
                 poseSpeed=3;
             end
        end
        
    % marsella, emotional gaze:
    % a+:faster move,body fw
%     if(vaFlag==1)
%         if( ar>50)%A+
%              poseSpeed=2;%high arouse fast move
%              poseLeanFlag=12;%high aroused lean fw
%         end
%         if(ar<-50)%A-
%              poseSpeed=3;%low arouse slow move
%              poseLeanFlag=11;%low aroused lean back
%         end
%     end 
    
    else%custom-flag==1
        poseFreqFactor=pose_frequency_custom;
        poseLean=pose_lean_custom;
        poseChanceFactor=pose_chance_custom;
        poseCatChance=pose_selfAdaptor_chance_custom;
        poseSpeed=pose_speed_custom;
    end

== matlab function Expriment_Pose/EmotionSubsystem/satFunction ==
  data: randv input; smile input; wave input; win input; invade input; v_trigW output; vaFlag input; v_trig output
function [v_trigW,v_trig]= fcn(randv,smile,wave,win,invade,vaFlag)
%#codegen
% 30/06/2015
    %Here set Agent's satisfaction flag based on your scenario
    %In RPS scenario agent gets satisfined when she wins. states of interaction= {STATE_READY=7;
    %STATE_GO=1;STATE_HAND=2;STATE_OVER=3; STATE_BEFORE=4;STATE_RESULT=5;STATE_WAIT=6;}
   
    if(vaFlag==1)
        v_trigW=0;%weight by which valence value is changed (sum of weight of all triggers)
        %randv 30% chance of random increase or decrease in valence
        randTrigger=floor(randv);
        if(0<randTrigger)&&(randTrigger<30)
            v_trigW = v_trigW + 0.6;
        end
        if(30<randTrigger)&&(randTrigger<60)
            v_trigW = v_trigW - 0.6;
        end

        if(win==2) %agent wins so she is satisfied
            v_trigW = v_trigW + 0.5;
        elseif(win==1) %user wins so agent is NOT satisfied
            v_trigW = v_trigW - 0.5;
        end

        if(smile==1)
            v_trigW=v_trigW+0.25;
        end

        if(wave==1)
            v_trigW=v_trigW+0.25;
        end

        if(invade==1)
            v_trigW=v_trigW-0.25;
        end
    else
         v_trigW=0;
    end
    if(v_trigW>0)
        v_trig=1;
    elseif(v_trigW<0)
        v_trig=-1;
        v_trigW=abs(v_trigW);
    else
        v_trig=0;
    end
